simulink model "magmantemplate15"  (R2015b)
settings: Solver=ode45  SolverMode=SingleTasking  StartTime=0.0  StopTime=30  FixedStep=h  RelTol=1e-3  AbsTol=1e-6
undefined symbols (not defined in the file or in its folder): Humusoft, MF634, sigbuilder_block
libraries: sldrtlib x1
settings Model: ExtModeTrigMode=oneshot  ExtModeArmWhenConnect=off  Creator=rbabuska  LastModifiedBy=rbabuska
settings DataIOCC: SaveFormat=Array  SignalLoggingSaveFormat=ModelDataLogs  SignalLoggingName=sigsOut
settings OptimizationCC: BooleanDataType=off  InitFltsAndDblsToZero=on
settings DebuggingCC: SaveWithParameterizedLinksMsg=none  UnderspecifiedInitializationDetection=Classic  MergeDetectMultiDrivingBlocksExec=none  SignalResolutionControl=TryResolveAllWithWarning  MultiTaskDSMMsg=warning  MultiTaskCondExecSysMsg=none  FcnCallInpInsideContextMsg=EnableAllAsWarning  AllowSymbolicDim=on
settings HardwareCC: ProdBitPerPointer=32  ProdLargestAtomicFloat=None  ProdIntDivRoundTo=Undefined  ProdEndianess=Unspecified  ProdWordSize=32  ProdHWDeviceType=32-bit Generic  TargetUnknown=on
settings GRTTargetCC: TargetFcnLib=ansi_tfl_tmw.mat  CombineOutputUpdateFcns=off  GRTInterface=on
settings ConfigComp: CovModelRefEnable=Off

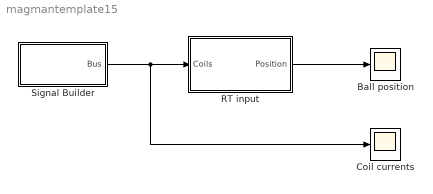
== system magmantemplate15 ==
  Ball position : Scope
  Coil currents : Scope
  RT input : Subsystem  mask{h=0.01, Port=['COM4';'COM5']}
      mask prompts: h "Sample time [s]:"; Port "Serial ports:"
      mask Display: disp('Magman')
  Signal Builder : Subsystem  Tag=STV Subsys  LoadFcn=sigbuilder_block('load');  StartFcn=sigbuilder_block('start');  StopFcn=sigbuilder_block('stop');  ClipboardFcn=sigbuilder_block('clipboard');  mask(Sigbuilder block){}
      mask help: Simulink:masks:SigbuilderBlock_MD
      mask init:
      | if ~strcmp(get_param(bdroot(gcbh),'SimulationStatus'),'stopped') tuvar = sigbuilder_block('maskInit'); end
      settings: CopyFcn=sigbuilder_block('copy');  DeleteFcn=sigbuilder_block('delete');  ModelCloseFcn=sigbuilder_block('modelClose');  PreSaveFcn=sigbuilder_block('preSave');  PauseFcn=sigbuilder_block('pause');  ContinueFcn=sigbuilder_block('continue');  NameChangeFcn=sigbuilder_block('namechange');  OpenFcn=sigbuilder_block('open',[437.6 199.2 550.4 400 ]);  CloseFcn=sigbuilder_block('close');
      mask Display: plot(0, 0, 100, 100,[2, 2, 32, 32, 2], [68, 8, 8, 68, 68],[32, 2], [38, 38], [32, 19, 2],[53, 60, 44], [32, 17, 17, 2],[16, 16, 31, 31]);txt = getActiveGroup(gcbh);text(2, 100, txt,'verticalAlignment', 'top');
  wires:
  Signal Builder/1(Bus) -> Coil currents/1, RT input/1(Coils)
  RT input/1(Position) -> Ball position/1

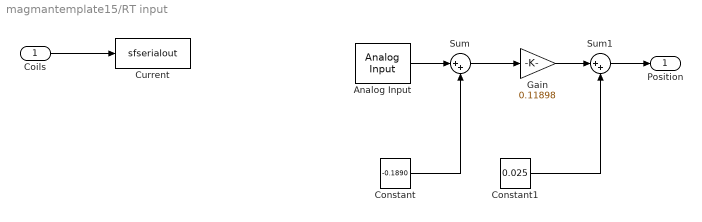
== system magmantemplate15/RT input ==
  Coils : Inport
  Analog Input : sldrtlib/Analog Input  SampleTime=h  MaxMissedTicks=100  ShowMissedTicks=off  YieldWhenWaiting=off  DrvName=Humusoft/MF634  DrvAddress=4294967295  DrvOptions=0  Channels=1  RangeMode=2  VoltRange=1  DataType=1
      settings: AttributesFormatString=Humusoft\nMF634 [auto]
  Constant : Constant  Value=-0.1890
  Constant1 : Constant  Value=0.025
  Current : S-Function  FunctionName=sfserialout  Parameters=h, com  SFunctionDeploymentMode=off  EnableBusSupport=off  mask(Serial Out){h=h, Port=Port}
      mask prompts: h "Sample time:"; Port "Serial port:"
      mask help: Serial line output block
      mask init:
      | com(1)              = rs232('GetParams','default'); % get default RS232 parameters
      | com(1).Port         = Port(1,:);                    % define port number
      | com(1).BaudRate     = 115200;                       % define Baud rate
      | com(1).ReadTimeout  = 1;                            % define short timeout
      | com(1).WriteTimeout = 1;                            % define short timeout
      | rs232('open',com(1));                               % open the port
      | 
      | com(2)              = rs232('GetParams','default'); % get default RS232 parameters
      | com(2).Port         = Port(2,:);                    % define port number
      | com(2).BaudRate     = 115200;                       % define Baud rate
      | com(2).ReadTimeout  = 1;                            % define short timeout
      | com(2).WriteTimeout = 1;                            % define short timeout
      | rs232('open',com(2)); 
      | 
      | %com(1) = serial(['COM' num2str(Port(1))],'BaudRate',115200,'Timeout',1,'DataBits',8,'StopBits',1,'Parity','none','Terminator','CR/LF');
      | %com(2) = serial(['COM' num2str(Port(2))],'BaudRate',115200,'Timeout',1,'DataBits',8,'StopBits',1,'Parity','none','Terminator','CR/LF');
      | %fopen(com);
      mask Help: Serial Out block is designed as a serial communication output block for real time data acquisition, signal processing and control applications.
      mask Display: disp('Coils');
  Gain : Gain  Gain=0.11898
  Sum : Sum  Inputs=|++
  Sum1 : Sum  Inputs=|++
  Position : Outport
  wires:
  Coils/1 -> Current/1
  Analog Input/1 -> Sum/1
  Constant/1 -> Sum/2
  Sum/1 -> Gain/1
  Gain/1 -> Sum1/1
  Sum1/1 -> Position/1
  Constant1/1 -> Sum1/2

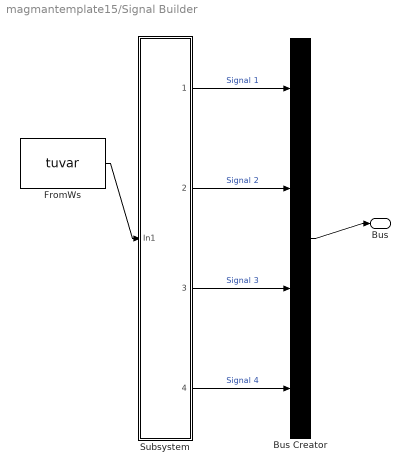
== system magmantemplate15/Signal Builder ==
  Bus Creator : BusCreator  Tag=Bus Creator  Inputs=4
  FromWs : FromWorkspace  Tag=STV FromWs  VariableName=tuvar  SampleTime=0
      SigBuilderData=|
      | common.afterFinalStr = 'Extrapolate'
      | common.sampleTime = 0
      | dataSet.timeRange = [0 30]
      | dataSet.name = 'Group 1'
      | sbobj.Groups.Name = 'Group 1'
      | sbobj.Groups.Signals(1).Name = 'Signal 1'
      | sbobj.Groups.Signals(1).XData = [0 5 5 10 30]
      | sbobj.Groups.Signals(1).YData = [0.6 0.6 -0.02 0 0]
      | sbobj.Groups.Signals(2).Name = 'Signal 2'
      | sbobj.Groups.Signals(2).XData = [0 4.05 4.05 11.9 11.9 30]
      | sbobj.Groups.Signals(2).YData = [0 0 0.6 0.6 0 0]
      | sbobj.Groups.Signals(3).Name = 'Signal 3'
      | sbobj.Groups.Signals(3).XData = [0 11 11 20 20 30]
      | sbobj.Groups.Signals(3).YData = [0 0 0.6 0.6 0 0]
      | sbobj.Groups.Signals(4).Name = 'Signal 4'
      | sbobj.Groups.Signals(4).XData = [0 18.85 18.85 30]
      | sbobj.Groups.Signals(4).YData = [0 0 0.6 0.6]
      | sbobj.Groups.TimeRange = [0 30]
  Subsystem : Subsystem
  Bus : Outport
  wires:
  FromWs/1 -> Subsystem/1(In1)
  Subsystem/1(Signal 1) -> Bus Creator/1  "Signal 1"
  Subsystem/2(Signal 2) -> Bus Creator/2  "Signal 2"
  Subsystem/3(Signal 3) -> Bus Creator/3  "Signal 3"
  Subsystem/4(Signal 4) -> Bus Creator/4  "Signal 4"
  Bus Creator/1 -> Bus/1

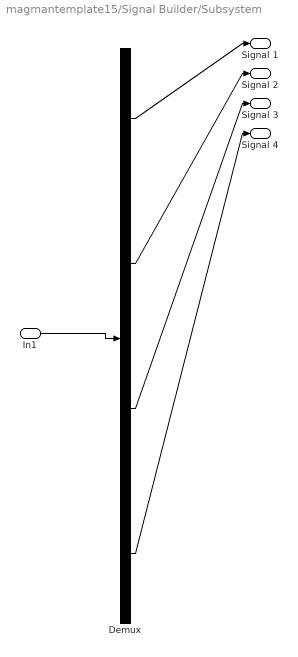
== system magmantemplate15/Signal Builder/Subsystem ==
  In1 : Inport
  Demux : Demux  Tag=STV Demux
  Signal 1 : Outport  Tag=STV Outport
  Signal 2 : Outport  Tag=STV Outport  Port=2
  Signal 3 : Outport  Tag=STV Outport  Port=3
  Signal 4 : Outport  Tag=STV Outport  Port=4
  wires:
  Demux/1 -> Signal 1/1
  Demux/2 -> Signal 2/1
  Demux/3 -> Signal 3/1
  Demux/4 -> Signal 4/1
  In1/1 -> Demux/1
